simulink model "sim_linear_control_error"  (R2018a)
settings: Solver=ode3  StartTime=0.0  StopTime=25  FixedStep=0.001  RelTol=1e-3
values from neighbouring files (symbols this model uses):
  A = [0         1                  0            0 ... (first row only)    [lin_control_error.m]    (also in lin_control_psi.m = [-(Cf+Cr)/(m*Vx)  -(a*Cf-b*Cr)/(m*Vx)-Vx; lin_control_y.m = [-(Cf+Cr)/(m*Vx)  -(a*Cf-b*Cr)/(m*Vx)-Vx; sys_compare.m = zeros(4,4))
  B = [0; 2*Cf/m; 0; 2*a*Cf/Iz]    [lin_control_error.m]    (also in lin_control_psi.m = [Cf/m; a*Cf/Iz]; lin_control_y.m = [Cf/m; a*Cf/Iz]; sys_compare.m = zeros(4,2))
  C = [0 1 0 0]    [lin_control_error.m]    (also in lin_control_psi.m = [0 1]; lin_control_y.m = [1 0])
  CA = C*A    [lin_control_error.m]    (also in lin_control_psi.m; lin_control_y.m)
  fc = 0.5    [lin_control_error.m]    (also in lin_control_y.m)
  G = [0; -2*(a*Cf-b*Cr)/(m*Vx)-Vx; 0; -2*(a^2*Cf+b^2*Cr)/(Iz*Vx)]    [lin_control_error.m]
  H = [0; 9.81; 0; 0]    [lin_control_error.m]
  invCB = pinv(C*B)    [lin_control_error.m]    (also in lin_control_psi.m; lin_control_y.m)
  Kb_e1 = 2    [lin_control_error.m]
  Kb_e1dot = 8    [lin_control_error.m]
  phi = 0    [lin_control_error.m]
  Vx = 30    [lin_control_error.m]    (also in lin_control_psi.m = 8.33333333333; lin_control_y.m = 8.33333333333)
  x0 = zeros(4,1)    [lin_control_error.m]
settings Model: Creator=E183308  LastModifiedBy=E183308

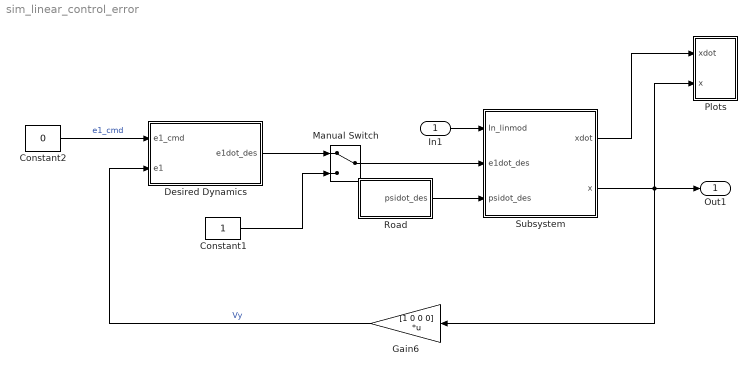
== system sim_linear_control_error ==
  In1 : Inport
  Constant1 : Constant
  Constant2 : Constant  Value=0
  Desired Dynamics : Subsystem
  Gain6 : Gain  Gain=[1 0 0 0]  Multiplication=Matrix(K*u)
  Manual Switch : ManualSwitch
  Plots : Subsystem
  Road : Subsystem
  Subsystem : Subsystem
  Out1 : Outport
  wires:
  Constant1/1 -> Manual Switch/2
  In1/1 -> Subsystem/1(In_linmod)
  Manual Switch/1 -> Subsystem/2(e1dot_des)
  Constant2/1 -> Desired Dynamics/1(e1_cmd)  "e1_cmd"
  Gain6/1 -> Desired Dynamics/2(e1)  "Vy"
  Desired Dynamics/1(e1dot_des) -> Manual Switch/1
  Subsystem/1(xdot) -> Plots/1(xdot)
  Subsystem/2(x) -> Gain6/1, Out1/1, Plots/2(x)
  Road/1(psidot_des) -> Subsystem/3(psidot_des)

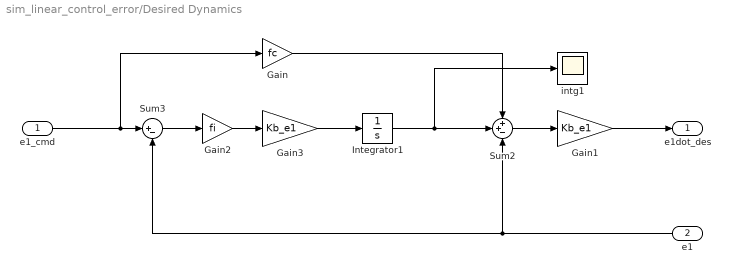
== system sim_linear_control_error/Desired Dynamics ==
  e1_cmd : Inport
  e1 : Inport  Port=2
  Gain : Gain  Gain=fc
  Gain1 : Gain  Gain=Kb_e1
  Gain2 : Gain  Gain=fi
  Gain3 : Gain  Gain=Kb_e1
  Integrator1 : Integrator
  Sum2 : Sum  Inputs=++-
  Sum3 : Sum  Inputs=|+-
  intg1 : Scope
  e1dot_des : Outport
  wires:
  Gain/1 -> Sum2/1
  Sum3/1 -> Gain2/1
  Gain3/1 -> Integrator1/1
  Integrator1/1 -> Sum2/2, intg1/1
  e1/1 -> Sum3/2, Sum2/3
  e1_cmd/1 -> Gain/1, Sum3/1
  Gain2/1 -> Gain3/1
  Gain1/1 -> e1dot_des/1
  Sum2/1 -> Gain1/1

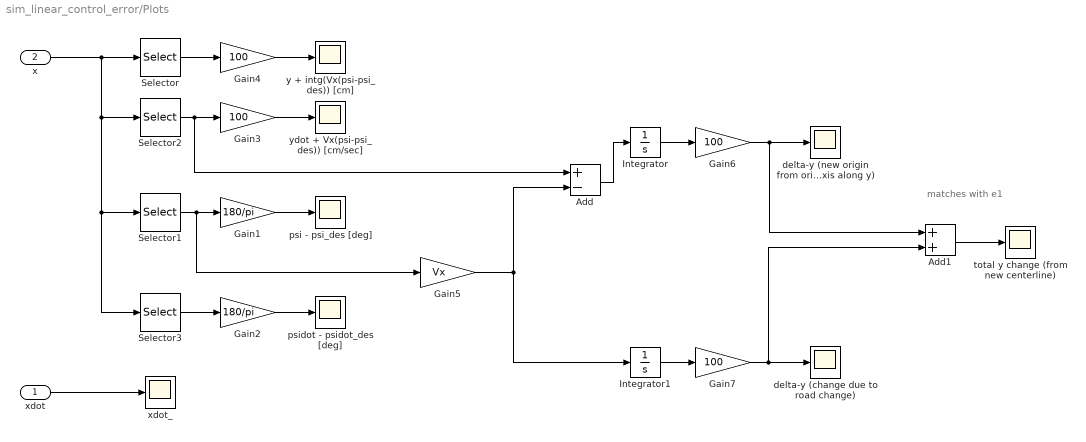
== system sim_linear_control_error/Plots ==
  note: matches with e1
  xdot : Inport
  x : Inport  Port=2
  Add : Sum  Inputs=+-
  Add1 : Sum
  Gain1 : Gain  Gain=180/pi
  Gain2 : Gain  Gain=180/pi
  Gain{3..4,6..7} (4 alike) : Gain  Gain=100
  Gain5 : Gain  Gain=Vx
  Integrator : Integrator
  Integrator1 : Integrator
  Selector : Selector  InputPortWidth=4  IndexOptions=Index vector (dialog)  Indices=1  OutputSizes=1
  Selector1 : Selector  InputPortWidth=4  IndexOptions=Index vector (dialog)  Indices=3  OutputSizes=1
  Selector2 : Selector  InputPortWidth=4  IndexOptions=Index vector (dialog)  Indices=2  OutputSizes=1
  Selector3 : Selector  InputPortWidth=4  IndexOptions=Index vector (dialog)  Indices=4  OutputSizes=1
  delta-y (change due to road change) : Scope
  delta-y (new origin from original axis along y) : Scope
  psi - psi_des [deg] : Scope
  psidot - psidot_des [deg] : Scope
  total y change (from new centerline) : Scope
  xdot_ : Scope
  y + intg(Vx(psi-psi_des)) [cm] : Scope
  ydot + Vx(psi-psi_des)) [cm/sec] : Scope
  wires:
  Selector1/1 -> Gain5/1, Gain1/1
  x/1 -> Selector2/1, Selector3/1, Selector1/1, Selector/1
  Selector/1 -> Gain4/1
  Gain1/1 -> psi - psi_des [deg]/1
  Gain4/1 -> y + intg(Vx(psi-psi_des)) [cm]/1
  xdot/1 -> xdot_/1
  Selector2/1 -> Add/1, Gain3/1
  Selector3/1 -> Gain2/1
  Gain2/1 -> psidot - psidot_des [deg]/1
  Gain3/1 -> ydot + Vx(psi-psi_des)) [cm/sec]/1
  Gain5/1 -> Add/2, Integrator1/1
  Add/1 -> Integrator/1
  Gain6/1 -> Add1/1, delta-y (new origin from original axis along y)/1
  Integrator/1 -> Gain6/1
  Integrator1/1 -> Gain7/1
  Gain7/1 -> Add1/2, delta-y (change due to road change)/1
  Add1/1 -> total y change (from new centerline)/1

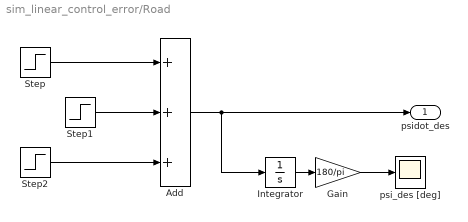
== system sim_linear_control_error/Road ==
  Add : Sum  Inputs=+++
  Gain : Gain  Gain=180/pi
  Integrator : Integrator
  Step : Step  Time=10  After=5*pi/180  SampleTime=0
  Step1 : Step  Time=13  After=-5*pi/180  SampleTime=0
  Step2 : Step  Time=16  After=5*pi/180*0  SampleTime=0
  psi_des [deg] : Scope
  psidot_des : Outport
  wires:
  Step/1 -> Add/1
  Step1/1 -> Add/2
  Step2/1 -> Add/3
  Add/1 -> Integrator/1, psidot_des/1
  Integrator/1 -> Gain/1
  Gain/1 -> psi_des [deg]/1

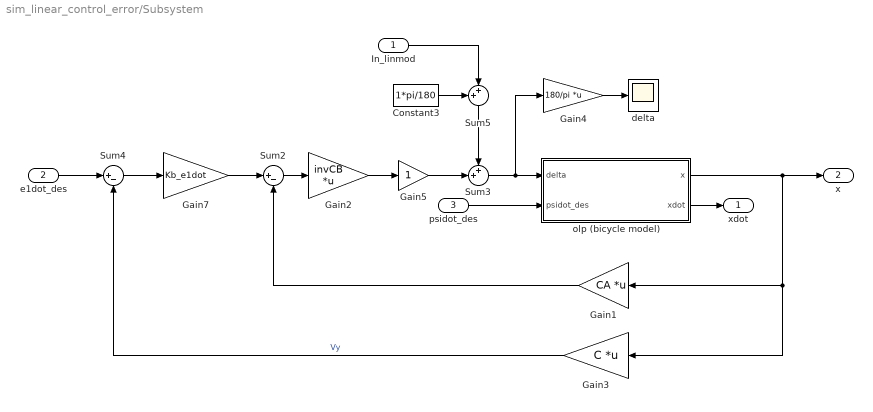
== system sim_linear_control_error/Subsystem ==
  In_linmod : Inport
  e1dot_des : Inport  Port=2
  psidot_des : Inport  Port=3
  Constant3 : Constant  Value=1*pi/180
  Gain1 : Gain  Gain=CA  Multiplication=Matrix(K*u)
  Gain2 : Gain  Gain=invCB  Multiplication=Matrix(K*u)
  Gain3 : Gain  Gain=C  Multiplication=Matrix(K*u)
  Gain4 : Gain  Gain=180/pi  Multiplication=Matrix(K*u)
  Gain5 : Gain
  Gain7 : Gain  Gain=Kb_e1dot
  Sum2 : Sum  Inputs=|+-
  Sum3 : Sum  Inputs=++|
  Sum4 : Sum  Inputs=|+-
  Sum5 : Sum  Inputs=++|
  delta : Scope
  olp (bicycle model) : Subsystem
  xdot : Outport
  x : Outport  Port=2
  wires:
  Gain4/1 -> delta/1
  e1dot_des/1 -> Sum4/1
  Gain3/1 -> Sum4/2  "Vy"
  Gain2/1 -> Gain5/1
  Sum2/1 -> Gain2/1
  Sum3/1 -> Gain4/1, olp (bicycle model)/1(delta)
  Sum4/1 -> Gain7/1
  Constant3/1 -> Sum5/1
  Sum5/1 -> Sum3/1
  Gain1/1 -> Sum2/2
  Gain7/1 -> Sum2/1
  In_linmod/1 -> Sum5/2
  olp (bicycle model)/1(x) -> Gain3/1, Gain1/1, x/1
  Gain5/1 -> Sum3/2
  olp (bicycle model)/2(xdot) -> xdot/1
  psidot_des/1 -> olp (bicycle model)/2(psidot_des)

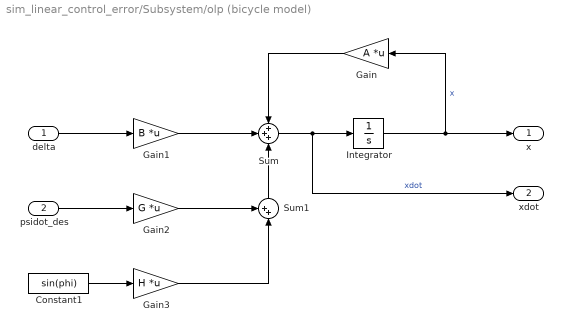
== system sim_linear_control_error/Subsystem/olp (bicycle model) ==
  delta : Inport
  psidot_des : Inport  Port=2
  Constant1 : Constant  Value=sin(phi)
  Gain : Gain  Gain=A  Multiplication=Matrix(K*u)
  Gain1 : Gain  Gain=B  Multiplication=Matrix(K*u)
  Gain2 : Gain  Gain=G  Multiplication=Matrix(K*u)
  Gain3 : Gain  Gain=H  Multiplication=Matrix(K*u)
  Integrator : Integrator  InitialCondition=x0
  Sum : Sum  Inputs=+++
  Sum1 : Sum  Inputs=++|
  x : Outport
  xdot : Outport  Port=2
  wires:
  Integrator/1 -> Gain/1, x/1  "x"
  delta/1 -> Gain1/1
  Sum/1 -> xdot/1, Integrator/1  "xdot"
  Gain/1 -> Sum/1
  Gain1/1 -> Sum/2
  psidot_des/1 -> Gain2/1
  Gain2/1 -> Sum1/1
  Sum1/1 -> Sum/3
  Constant1/1 -> Gain3/1
  Gain3/1 -> Sum1/2
